simulink subsystem "Spieleecke"  (R2022b)
settings: Solver=VariableStepAuto  StartTime=0.0  StopTime=10.0  RelTol=1e-3
settings Model: LastModifiedBy=timos
settings OptimizationCC: ReuseModelBlockBuffer=on
settings RTWCC: GPUComputeCapability=5.0
settings ConfigComp: CovBoundaryAbsTol=1.0e-5

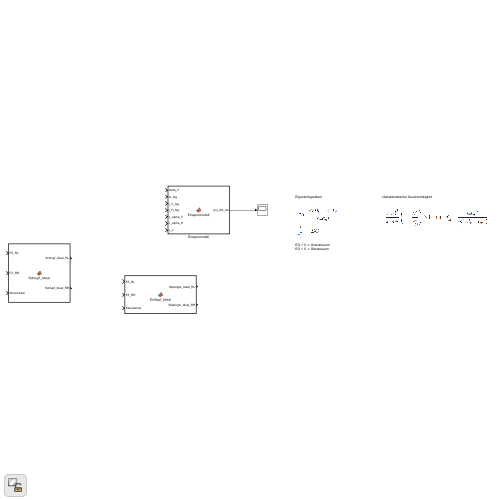
[thumbnail: Simulink's stored preview of the top-level diagram]
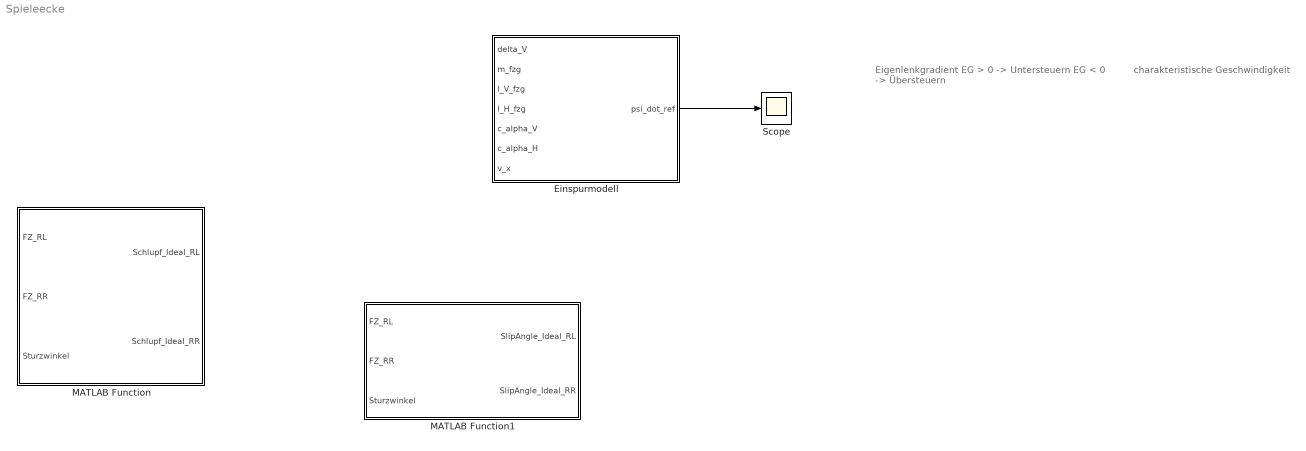
== system Spieleecke ==
  note: Eigenlenkgradient
      |
      | EG > 0 -> Untersteuern
      | EG < 0 -> Übersteuern
  note: charakteristische Geschwindigkeit
  Einspurmodell : MATLAB Function  TreatAsAtomicUnit=on
  MATLAB Function : MATLAB Function  TreatAsAtomicUnit=on
  MATLAB Function1 : MATLAB Function  TreatAsAtomicUnit=on
  Scope : Scope
  wires:
  Einspurmodell/1(psi_dot_ref) -> Scope/1

== matlab function Spieleecke/Einspurmodell ==
  data: psi_dot_ref output; delta_V input; m_fzg input; l_V_fzg input; l_H_fzg input; c_alpha_V input; c_alpha_H input; v_x input
function psi_dot_ref  = Einspurmodell(delta_V, m_fzg, l_V_fzg, l_H_fzg, c_alpha_V, c_alpha_H, v_x)
%#codegen

% Charakteristische Geschwindigkeit zum Quadrat
square_v_ch = c_alpha_V * c_alpha_H * l_fzg / (m_fzg * ((c_alpha_H * l_H_fzg) - (c_alpha_V * l_V_fzg)));

% Soll Gierrate
psi_dot_ref = v_x * delta_V / (l_fzg * (1 + (v_x^2 / square_v_ch)));
end

== matlab function Spieleecke/MATLAB Function ==
  data: FZ_RL input; Schlupf_Ideal_RL output; FZ_RR input; Sturzwinkel input; Schlupf_Ideal_RR output
function [Schlupf_Ideal_RL,Schlupf_Ideal_RR] = Schlupf_Ideal(FZ_RL,FZ_RR,Sturzwinkel)
% =======================================================================
% Magic Formula Parameter
% Scaling und Shape Koeffizienten
LCX   				= 1;
LMUX  				= 0.75;
LEX   				= 1;
LKX   				= 1;
LHX   				= 1;
LVX   				= 1;
LGAX  				= 1;
% Longitudinal Koeffizienten
PCX1  				= +1.786E+000;
PDX1  				= +2.688E+000;
PDX2  				= -2.720E-001;
PDX3  				= +1.370E+001;
PEX1  				= +8.710E-001;
PEX2  				= -3.800E-002;
PEX3  				= +0.000E+000;
PEX4  				= +7.100E-002;
PKX1  				= +8.125E+001;
PKX2  				= -2.025E+001;
PKX3  				= +5.000E-001;
PHX1  				= +0.000E+000;
PHX2  				= +0.000E+000;
PVX1  				= +0.000E+000;
PVX2  				= +0.000E+000;
% =======================================================================
% RL
i = 0;
Fz = FZ_RL;
GAMMA = Sturzwinkel;
FX_RL = zeros((0.3/0.01),3);                                                % Vorinitialisierung
for KAPPA = 0:0.01:0.3
    % ====================================================================
    % Magic Formula Berechnung FX // Nur Längsschlupf
    GAMMAX = GAMMA .* LGAX;
    SHX = (PHX1 + PHX2 .* DFZ) .* LHX;
    KAPPAX = KAPPA + SHX;
    CX = PCX1 .* LCX;
    MUX = (PDX1 + PDX2 .* DFZ) .* (1 - PDX3 .* GAMMAX.^2) .* LMUX;
    DX = MUX .* Fz;
    EX = (PEX1 + PEX2 .* DFZ + PEX3 .* DFZ.^2) .* (1 - PEX4 .* sign(KAPPAX)) .* LEX;
    KX = Fz .* (PKX1 + PKX2 .* DFZ) .* exp(PKX3 .* DFZ) .* LKX;
    BX = KX ./ (CX .* DX);
    SVX = Fz .* (PVX1 + PVX2 .* DFZ) .* LVX .* LMUX;
    % ====================================================================
    % Eintragung in die Matrix
    i=i+1;
    FX_RL(i,1) = Fz;
    FX_RL(i,2) = KAPPA;
    FX_RL(i,3) = DX .* sin(CX .* atan(BX .* KAPPAX - EX .* (BX .* KAPPAX - atan(BX .* KAPPAX)))) + SVX;
end
[~, Index] = max(FX_RL(:,3));                                               % Zeilennummer des maximalen FX-Werte
Schlupf_Ideal_RL = FX_RL(Index,:);                                          % Eintragung in die Ausgabegröße
% =======================================================================
% RR
i = 0;
Fz = FZ_RR;
GAMMA = Sturzwinkel;
FX_RR = zeros((0.3/0.01),3);                                                % Vorinitialisierung
for KAPPA = 0:0.01:0.3
    % ====================================================================
    % Magic Formula Berechnung FX // Nur Längsschlupf
    GAMMAX = GAMMA .* LGAX;
    SHX = (PHX1 + PHX2 .* DFZ) .* LHX;
    KAPPAX = KAPPA + SHX;
    CX = PCX1 .* LCX;
    MUX = (PDX1 + PDX2 .* DFZ) .* (1 - PDX3 .* GAMMAX.^2) .* LMUX;
    DX = MUX .* Fz;
    EX = (PEX1 + PEX2 .* DFZ + PEX3 .* DFZ.^2) .* (1 - PEX4 .* sign(KAPPAX)) .* LEX;
    KX = Fz .* (PKX1 + PKX2 .* DFZ) .* exp(PKX3 .* DFZ) .* LKX;
    BX = KX ./ (CX .* DX);
    SVX = Fz .* (PVX1 + PVX2 .* DFZ) .* LVX .* LMUX;
    % ====================================================================
    % Eintragung in die Matrix
    i=i+1;
    FX_RR(i,1) = Fz;
    FX_RR(i,2) = KAPPA;
    FX_RR(i,3) = DX .* sin(CX .* atan(BX .* KAPPAX - EX .* (BX .* KAPPAX - atan(BX .* KAPPAX)))) + SVX;
end
[~, Index] = max(FX_RR(:,3));                                               % Zeilennummer des maximalen FX-Werte
Schlupf_Ideal_RR = FX_RR(Index,:);                                          % Eintragung in die Ausgabegröße

== matlab function Spieleecke/MATLAB Function1 ==
  data: FZ_RL input; SlipAngle_Ideal_RL output; FZ_RR input; Sturzwinkel input; SlipAngle_Ideal_RR output
function [SlipAngle_Ideal_RL,SlipAngle_Ideal_RR] = Schlupf_Ideal(FZ_RL,FZ_RR,Sturzwinkel)
% Scaling und Shape Koeffizienten
LCY   				= 0.90;
LMUY  				= 0.75;
LEY   				= 1;
LKY   				= 1;
LHY   				= 0;
LVY   				= 0;
LGAY  				= 0.75;
% Laterale Koeffizienten
PCY1				= +1.625E+000;
PDY1				= +2.554E+000;
PDY2				= -4.021E-001;
PDY3				= +5.406E+000;
PEY1				= +1.715E-001;
PEY2				= -8.339E-001;
PEY3				= -1.743E-001;
PEY4				= -6.110E+000;
PKY1				= -5.912E+001;
PKY2				= +2.567E+000;
PKY3				= +4.787E-001;
PHY1				= +0.000E+000;
PHY2				= +0.000E+000;
PHY3				= -2.152E-002;
PVY1				= +0.000E+000;
PVY2				= +0.000E+000;
PVY3				= -2.151E+000;
PVY4				= -8.772E-001;
% =======================================================================
% RL
i = 0;
Fz = FZ_RL;
GAMMA = Sturzwinkel;
FY_RL = zeros((12/0.1),3);                                                  % Vorinitialisierung
for ALPHA = 0:0.1:12
    % ====================================================================
    % Magic Formula Berechnung FX // Nur Längsschlupf
    GAMMAY = GAMMA .* LGAY;
    SHY = (PHY1 + PHY2 .* DFZ) .* LHY + PHY3 .* GAMMAY;
    ALPHAY = ALPHA + SHY;
    CY = PCY1 .* LCY;
    MUY = (PDY1 + PDY2 .* DFZ) .* (1 - PDY3 .* GAMMAY.^2) .* LMUY;
    DY = MUY .* Fz;
    EY = (PEY1 + PEY2 .* DFZ) .* (1 - (PEY3 + PEY4 .* GAMMAY) .* sign(ALPHAY)) .* LEY;
    KY = PKY1 .* FZ0 .* sin(2 * atan(Fz ./ (PKY2 .* FZ0 .* LFZO))) .* (1 - PKY3 .* abs(GAMMAY)) .* LFZO .* LKY;
    BY = KY ./ (CY .* DY);
    SVY = Fz .* ((PVY1 + PVY2 .* DFZ) .* LVY + (PVY3 + PVY4 .* DFZ) .* GAMMAY) .* LMUY;
    % ====================================================================
    % Eintragung in die Matrix
    i=i+1;
    FY_RL(i,1) = Fz;
    FY_RL(i,2) = ALPHA;
    FY_RL(i,3) = DY .* sin(CY .* atan(BY .* ALPHAY - EY .* (BY .* ALPHAY - atan(BY .* ALPHAY)))) + SVY;
end
[~, Index] = max(FY_RL(:,3));                                               % Zeilennummer des maximalen FX-Werte
SlipAngle_Ideal_RL = FY_RL(Index,2);                                        % Eintragung in die Ausgabegröße
% =======================================================================
% RR
i = 0;
Fz = FZ_RR;
GAMMA = Sturzwinkel;
FY_RR = zeros((12/0.1),3);                                                  % Vorinitialisierung
for ALPHA = 0:0.1:12
    % ====================================================================
    % Magic Formula Berechnung FX // Nur Längsschlupf
    GAMMAY = GAMMA .* LGAY;
    SHY = (PHY1 + PHY2 .* DFZ) .* LHY + PHY3 .* GAMMAY;
    ALPHAY = ALPHA + SHY;
    CY = PCY1 .* LCY;
    MUY = (PDY1 + PDY2 .* DFZ) .* (1 - PDY3 .* GAMMAY.^2) .* LMUY;
    DY = MUY .* Fz;
    EY = (PEY1 + PEY2 .* DFZ) .* (1 - (PEY3 + PEY4 .* GAMMAY) .* sign(ALPHAY)) .* LEY;
    KY = PKY1 .* FZ0 .* sin(2 * atan(Fz ./ (PKY2 .* FZ0 .* LFZO))) .* (1 - PKY3 .* abs(GAMMAY)) .* LFZO .* LKY;
    BY = KY ./ (CY .* DY);
    SVY = Fz .* ((PVY1 + PVY2 .* DFZ) .* LVY + (PVY3 + PVY4 .* DFZ) .* GAMMAY) .* LMUY;
    % ====================================================================
    % Eintragung in die Matrix
    i=i+1;
    FY_RR(i,1) = Fz;
    FY_RR(i,2) = ALPHA;
    FY_RR(i,3) = DY .* sin(CY .* atan(BY .* ALPHAY - EY .* (BY .* ALPHAY - atan(BY .* ALPHAY)))) + SVY;
end
[~, Index] = max(FY_RR(:,3));                                               % Zeilennummer des maximalen FX-Werte
SlipAngle_Ideal_RR = FY_RR(Index,2);                                        % Eintragung in die Ausgabegröße
